simulink model "three_phase_inv"  (R2024a)
settings: Solver=VariableStepAuto  StartTime=0.0  StopTime=0.1  MaxStep=1e-6  RelTol=1e-3
values from neighbouring files (symbols this model uses):
  filter_capacitance = 1e-3    (= 0.001)    [constants.m]
  filter_inductance = 1e-5    (= 1e-05)    [constants.m]
  m_index = 1    [constants.m]
libraries: spsGroundLib x13, spsMosfetLib x6, spsVoltageMeasurementLib x6, spsParallelRLCBranchLib x4, simulink x3, spsSeriesRLCBranchLib x3, spsDCVoltageSourceLib x1, spsTriangleGeneratorLib x1, sps_lib x1
settings Model: Creator=RASM  LastModifiedBy=RASM

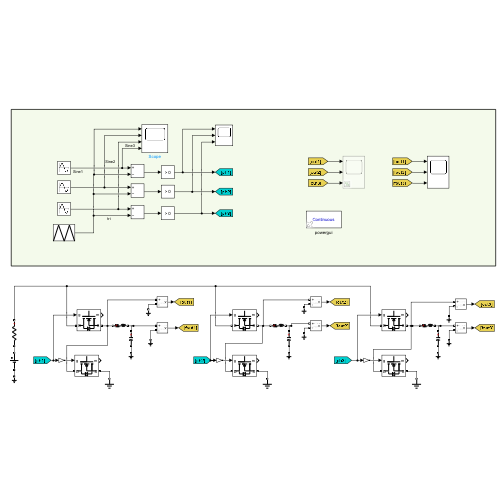
[thumbnail: Simulink's stored preview of the top-level diagram]
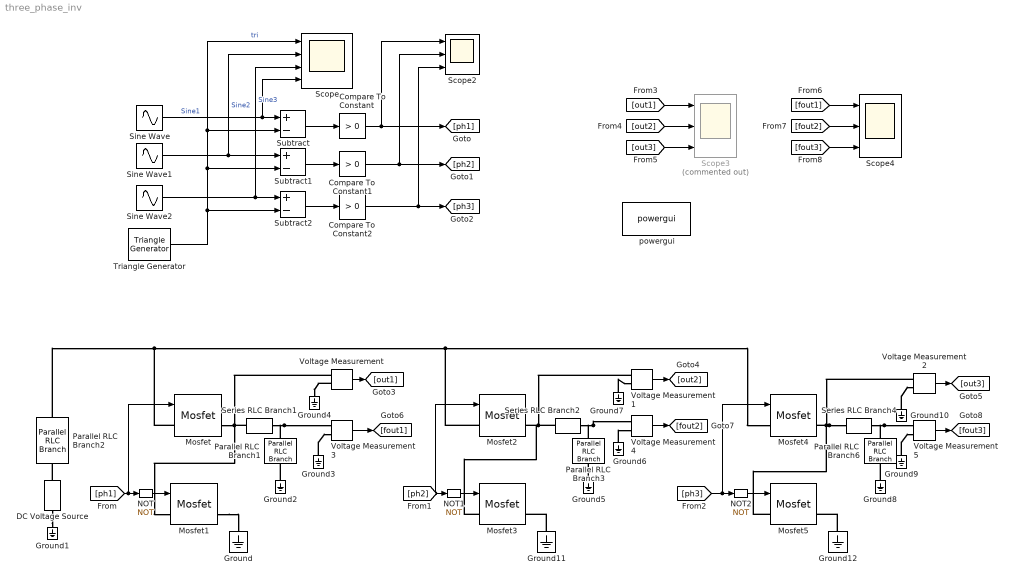
== system three_phase_inv ==
  Compare To Constant : simulink/Logic and Bit Operations/Compare To Constant  relop=>  const=0  OutDataTypeStr=boolean
  Compare To Constant1 : simulink/Logic and Bit Operations/Compare To Constant  relop=>  const=0  OutDataTypeStr=boolean
  Compare To Constant2 : simulink/Logic and Bit Operations/Compare To Constant  relop=>  const=0  OutDataTypeStr=boolean
  DC Voltage Source : spsDCVoltageSourceLib/DC Voltage Source  Amplitude=12  Measurements=None
  Ground{,1..12} (13 alike) : spsGroundLib/Ground  LConnTagsString=a
  Mosfet{,1..5} (6 alike) : spsMosfetLib/Mosfet  Ron=0.1  Lon=0  Rd=0.01  Vfd=0  IC=0  Rs=1e5  Cs=inf  Measurements=on
  NOT : Logic  Operator=NOT  IconShape=distinctive  AllPortsSameDT=off  OutDataTypeStr=boolean
  NOT1 : Logic  Operator=NOT  IconShape=distinctive  AllPortsSameDT=off  OutDataTypeStr=boolean
  NOT2 : Logic  Operator=NOT  IconShape=distinctive  AllPortsSameDT=off  OutDataTypeStr=boolean
  Parallel RLC Branch1 : spsParallelRLCBranchLib/Parallel RLC Branch  LConnTagsString=a  RConnTagsString=__new0  BranchType=C  Resistance=10  Inductance=filter_inductance  SetiL0=off  InitialCurrent=0  Capacitance=filter_capacitance  Setx0=off  InitialVoltage=0  Measurements=None
  Parallel RLC Branch2 : spsParallelRLCBranchLib/Parallel RLC Branch  LConnTagsString=a  RConnTagsString=__new0  BranchType=R  Resistance=0.1  Inductance=filter_inductance  SetiL0=off  InitialCurrent=0  Capacitance=1e-6  Setx0=off  InitialVoltage=0  Measurements=None
  Parallel RLC Branch3 : spsParallelRLCBranchLib/Parallel RLC Branch  LConnTagsString=a  RConnTagsString=__new0  BranchType=C  Resistance=10  Inductance=filter_inductance  SetiL0=off  InitialCurrent=0  Capacitance=filter_capacitance  Setx0=off  InitialVoltage=0  Measurements=None
  Parallel RLC Branch6 : spsParallelRLCBranchLib/Parallel RLC Branch  LConnTagsString=a  RConnTagsString=__new0  BranchType=C  Resistance=10  Inductance=filter_inductance  SetiL0=off  InitialCurrent=0  Capacitance=filter_capacitance  Setx0=off  InitialVoltage=0  Measurements=None
  Scope : Scope  NumInputPorts=4
  Scope2 : Scope  NumInputPorts=3
  Scope3 : Scope  Commented=on  NumInputPorts=3
  Scope4 : Scope  NumInputPorts=3
  Series RLC Branch1 : spsSeriesRLCBranchLib/Series RLC Branch  LConnTagsString=__new0  RConnTagsString=__new0  BranchType=RL  Resistance=1e-3  Inductance=filter_inductance  SetiL0=off  InitialCurrent=0  Capacitance=0  Setx0=off  InitialVoltage=0  Measurements=None
  Series RLC Branch2 : spsSeriesRLCBranchLib/Series RLC Branch  LConnTagsString=__new0  RConnTagsString=__new0  BranchType=RL  Resistance=1e-3  Inductance=filter_inductance  SetiL0=off  InitialCurrent=0  Capacitance=0  Setx0=off  InitialVoltage=0  Measurements=None
  Series RLC Branch4 : spsSeriesRLCBranchLib/Series RLC Branch  LConnTagsString=__new0  RConnTagsString=__new0  BranchType=RL  Resistance=1e-3  Inductance=filter_inductance  SetiL0=off  InitialCurrent=0  Capacitance=0  Setx0=off  InitialVoltage=0  Measurements=None
  Sine Wave : Sin  Amplitude=1 * m_index  Frequency=2*pi*50  Phase=(4*pi)/3  SampleTime=0
  Sine Wave1 : Sin  Amplitude=1 * m_index  Frequency=2*pi*50  Phase=(2*pi)/3  SampleTime=0
  Sine Wave2 : Sin  Amplitude=1 * m_index  Frequency=2*pi*50  SampleTime=0
  Subtract : Sum  Inputs=+-
  Subtract1 : Sum  Inputs=+-
  Subtract2 : Sum  Inputs=+-
  Triangle Generator : spsTriangleGeneratorLib/Triangle Generator  Freq=freq_m  Phase=0  Ts=0
  Voltage Measurement{,1..5} (6 alike) : spsVoltageMeasurementLib/Voltage Measurement  PhasorSimulation=off  OutputType=Complex  PSBequivalent=0
  powergui : sps_lib/powergui  Priority=1  SimulationMode=Continuous  SampleTime=50e-6  frequency=50  Iterations=50  frequencyindice=0  Pbase=100e6  ErrMax=1e-4  UnitsV=kV  UnitsW=MW  buscounter=0  FunctionMessages=off  echomessages=off  EnableUseOfTLC=off  CurrentSourceSwitches=off  DisableSnubberDevices=off  DisableRonSwitches=off  DisableVfSwitches=off  DisplayEquations=off  AutomaticDiscreteSolvers=off  SolverType=Tustin/Backward Euler (TBE)  Interpol=off  ExternalGateDelay=off  methode=off  Ts=100  x0status=blocks  SPID=on  SwTol=0  HookPort=off  NonlinearTolerance=1e-4  nMaxIteration=100  ContinueOnMaxIteration=off  RestoreLinks=warning  ResistiveCurrentMeasurement=off  Frange=[0:2:500]  Ylog=off  Xlog=on  ShowGrid=off  save=off  variable=ZData  structure=0  ZoomFFT=off  StartTime=0.0  cycles=1  DisplayStyle=1  fundamental=60  FreqAxis=off  MaxFrequency=1000  frequencyindicesteady=1  RmsSteady=1  display=off
  wires:
  Sine Wave/1 -> Scope/4, Subtract/1  "Sine1"
  Subtract/1 -> Compare To Constant/1
  Subtract1/1 -> Compare To Constant1/1
  Sine Wave1/1 -> Subtract1/1, Scope/2  "Sine2"
  Sine Wave2/1 -> Subtract2/1, Scope/3  "Sine3"
  Subtract2/1 -> Compare To Constant2/1
  Triangle Generator/1 -> Subtract2/2, Subtract1/2, Scope/1, Subtract/2  "tri"
  Compare To Constant2/1 -> [ph3], Scope2/3
  Compare To Constant1/1 -> [ph2], Scope2/2
  Compare To Constant/1 -> [ph1], Scope2/1
  NOT/1 -> Mosfet1/1
  NOT1/1 -> Mosfet3/1
  NOT2/1 -> Mosfet5/1
  [ph1] -> Mosfet/1, NOT/1
  [ph2] -> Mosfet2/1, NOT1/1
  [ph3] -> Mosfet4/1, NOT2/1
  Voltage Measurement/1 -> [out1]
  [out1] -> Scope3/1
  Voltage Measurement1/1 -> [out2]
  [out2] -> Scope3/2
  Voltage Measurement2/1 -> [out3]
  [out3] -> Scope3/3
  Voltage Measurement3/1 -> [fout1]
  Voltage Measurement4/1 -> [fout2]
  Voltage Measurement5/1 -> [fout3]
  [fout3] -> Scope4/3
  [fout2] -> Scope4/2
  [fout1] -> Scope4/1
  connections:
  Mosfet/LConn1 -- Mosfet2/LConn1 -- Mosfet4/LConn1 -- Parallel RLC Branch2/LConn1
  DC Voltage Source/LConn1 -- Ground1/LConn1
  Voltage Measurement/LConn2 -- Ground4/LConn1
  Ground7/LConn1 -- Voltage Measurement1/LConn2
  Ground10/LConn1 -- Voltage Measurement2/LConn2
  Ground3/LConn1 -- Voltage Measurement3/LConn2
  Ground6/LConn1 -- Voltage Measurement4/LConn2
  Ground9/LConn1 -- Voltage Measurement5/LConn2
  DC Voltage Source/RConn1 -- Parallel RLC Branch2/RConn1
  Mosfet/RConn1 -- Series RLC Branch1/LConn1 -- Voltage Measurement/LConn1 -- Mosfet1/LConn1
  Mosfet3/LConn1 -- Series RLC Branch2/LConn1 -- Voltage Measurement1/LConn1 -- Mosfet2/RConn1
  Parallel RLC Branch6/LConn1 -- Series RLC Branch4/RConn1 -- Voltage Measurement5/LConn1
  Ground8/LConn1 -- Parallel RLC Branch6/RConn1
  Mosfet5/LConn1 -- Series RLC Branch4/LConn1 -- Mosfet4/RConn1 -- Voltage Measurement2/LConn1
  Parallel RLC Branch3/LConn1 -- Series RLC Branch2/RConn1 -- Voltage Measurement4/LConn1
  Ground5/LConn1 -- Parallel RLC Branch3/RConn1
  Parallel RLC Branch1/LConn1 -- Series RLC Branch1/RConn1 -- Voltage Measurement3/LConn1
  Ground2/LConn1 -- Parallel RLC Branch1/RConn1
  Mosfet1/RConn1 -- Ground/LConn1
  Ground11/LConn1 -- Mosfet3/RConn1
  Ground12/LConn1 -- Mosfet5/RConn1
